simulink model "modelo_ident"  (R2023b)
settings: Solver=ode45  StartTime=0.0  StopTime=5000  RelTol=1e-3  EnableMultiTasking=on
undefined symbols (not defined in the file): Ts
libraries: simulink x2
settings Model: Creator=Electronica  LastModifiedBy=juanj
settings SolverCC: AlgebraicLoopSolver=TrustRegion
settings DataIOCC: LimitDataPoints=on  SaveFormat=Array  ReturnWorkspaceOutputs=off
settings OptimizationCC: LifeSpan=inf
settings DebuggingCC: UnderspecifiedInitializationDetection=Classic  MergeDetectMultiDrivingBlocksExec=none  SolverPrmCheckMsg=warning  UnconnectedInputMsg=warning  UnconnectedOutputMsg=warning  UnconnectedLineMsg=warning  StateNameClashWarn=warning  SFUnexpectedBacktrackingDiag=warning  SFNoUnconditionalDefaultTransitionDiag=warning  ArithmeticOperatorsInVariantConditions=warning
settings HardwareCC: ProdBitPerPointer=32  ProdBitPerSizeT=32  ProdBitPerPtrDiffT=32  ProdLargestAtomicFloat=None  ProdIntDivRoundTo=Undefined  ProdEndianess=Unspecified  ProdWordSize=32  ProdHWDeviceType=32-bit Generic
settings ModelReferenceCC: EnableRefExpFcnMdlSchedulingChecks=on  PropagateSignalLabelsOutOfModel=off
settings SFSimCC: SimUseLocalCustomCode=off  CustomCodeUndefinedFunction=UseInterfaceOnly
settings RTWCC: RTWUseLocalCustomCode=off
settings CodeAppCC: StateflowObjectComments=on
settings GRTTargetCC: TargetLangStandard=C89/C90 (ANSI)
settings ConfigComp: CovMetricSettings=dw  CovSaveCumulativeToWorkspaceVar=on  CovSaveSingleToWorkspaceVar=on  CovExternalEMLEnable=off

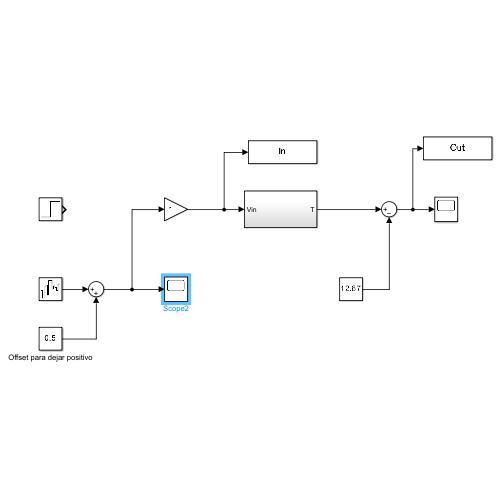
[thumbnail: Simulink's stored preview of the top-level diagram]
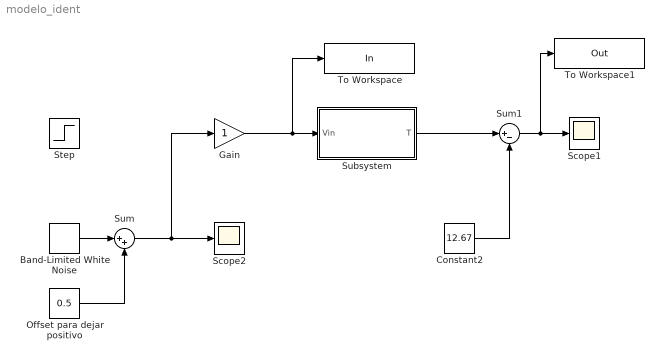
== system modelo_ident ==
  Band-Limited White Noise : simulink/Sources/Band-Limited White Noise  Cov=[0.4]*8  Ts=Ts  seed=[23341]
  Constant2 : Constant  Value=12.67
  Gain : Gain
  Offset para dejar positivo : Constant  Value=0.5
  Scope1 : Scope
  Scope2 : Scope
  Step : Step  Time=0  After=5  SampleTime=0
  Subsystem : Subsystem
  Sum : Sum  Inputs=|++
  Sum1 : Sum  Inputs=|+-
  To Workspace : ToWorkspace  VariableName=In  SampleTime=Ts
  To Workspace1 : ToWorkspace  VariableName=Out  SampleTime=Ts
  wires:
  Sum/1 -> Gain/1, Scope2/1
  Subsystem/1(T) -> Sum1/1
  Sum1/1 -> To Workspace1/1, Scope1/1
  Gain/1 -> To Workspace/1, Subsystem/1(Vin)
  Band-Limited White Noise/1 -> Sum/1
  Offset para dejar positivo/1 -> Sum/2
  Constant2/1 -> Sum1/2

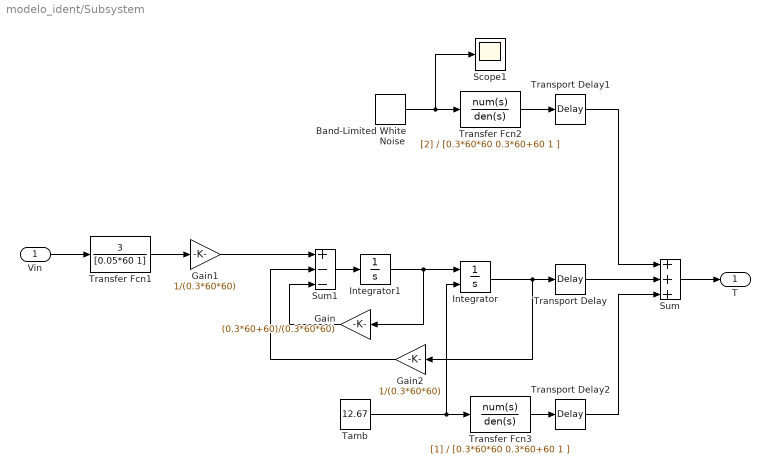
== system modelo_ident/Subsystem ==
  Vin : Inport
  Band-Limited White Noise : simulink/Sources/Band-Limited White Noise  Cov=[0.1]  Ts=18  seed=[23341]
  Gain : Gain  Gain=(0.3*60+60)/(0.3*60*60)
  Gain1 : Gain  Gain=1/(0.3*60*60)
  Gain2 : Gain  Gain=1/(0.3*60*60)
  Integrator : Integrator  InitialConditionSource=external
  Integrator1 : Integrator
  Scope1 : Scope
  Sum : Sum  Inputs=+++
  Sum1 : Sum  Inputs=+--
  "Tamb " : Constant  Value=12.67
  Transfer Fcn1 : TransferFcn  Numerator=[3]  Denominator=[0.05*60 1]
  Transfer Fcn2 : TransferFcn  Numerator=[2]  Denominator=[0.3*60*60 0.3*60+60 1 ]
  Transfer Fcn3 : TransferFcn  Denominator=[0.3*60*60 0.3*60+60 1 ]
  Transport Delay : TransportDelay  DelayTime=0.1*60  InitialOutput=12.67
  Transport Delay1 : TransportDelay  DelayTime=0.1*60
  Transport Delay2 : TransportDelay  DelayTime=0.1*60
  T : Outport
  wires:
  Transfer Fcn1/1 -> Gain1/1
  Integrator/1 -> Transport Delay/1, Gain2/1
  Sum/1 -> T/1
  Transfer Fcn2/1 -> Transport Delay1/1
  Band-Limited White Noise/1 -> Scope1/1, Transfer Fcn2/1
  Transport Delay1/1 -> Sum/1
  Transfer Fcn3/1 -> Transport Delay2/1
  Transport Delay2/1 -> Sum/3
  Gain1/1 -> Sum1/1
  Gain/1 -> Sum1/3
  Gain2/1 -> Sum1/2
  "Tamb "/1 -> Integrator/2, Transfer Fcn3/1
  Integrator1/1 -> Integrator/1, Gain/1
  Sum1/1 -> Integrator1/1
  Transport Delay/1 -> Sum/2
  Vin/1 -> Transfer Fcn1/1
